simulink model "USV_SASTnewlaw_env_max"  (R2023a)
settings: Solver=ode4  StartTime=0.0  StopTime=60  FixedStep=0.01  RelTol=1e-3
undefined symbols (not defined in the file or in its folder): sigbuilder_block
libraries: sharedutil x6, simulink_extras x1, aerolibutil x1
(part 2 of 2)

== system USV_SASTnewlaw_env_max/USV_Env/Dynamic Model/Construct Matrices/M ==
  m : Inport
  X_G : Inport  Port=2
  Y_G : Inport  Port=3
  I_z : Inport  Port=4
  Hydrodynamic coefficients : Inport  Port=5
  Bus Selector : BusSelector  OutputSignals=X_u_dot,Y_r_dot,N_v_dot,Y_v_dot,N_r_dot
  Constant3 : Constant  Value=0
  Gain8 : Gain  Gain=-1
  Matrix M : sharedutil/Create 3x3 Matrix  aMode=aMode
  Product17 : Product
  Product18 : Product
  Sum14 : Sum  Inputs=|+-
  Sum15 : Sum  Inputs=+-
  Sum16 : Sum  Inputs=+-
  Sum17 : Sum  Inputs=+-
  Sum18 : Sum  Inputs=|+-
  M : Outport  VectorParamsAs1DForOutWhenUnconnected=off
  wires:
  Gain8/1 -> Matrix M/7, Matrix M/3
  Product17/1 -> Gain8/1
  Product18/1 -> Sum17/1, Sum16/1
  Sum18/1 -> Matrix M/9
  Constant3/1 -> Matrix M/4, Matrix M/2
  I_z/1 -> Sum18/1  "I_z"
  Sum15/1 -> Matrix M/5
  m/1 -> Sum14/1, Product17/1, Sum15/1, Product18/1  "m"
  Bus Selector/3 -> Sum17/2  "<N_v_dot>"
  Sum14/1 -> Matrix M/1
  Sum16/1 -> Matrix M/6
  Matrix M/1 -> M/1
  Sum17/1 -> Matrix M/8
  X_G/1 -> Product18/2  "X_G"
  Y_G/1 -> Product17/2  "Y_G"
  Bus Selector/1 -> Sum14/2  "<X_u_dot>"
  Hydrodynamic coefficients/1 -> Bus Selector/1
  Bus Selector/2 -> Sum16/2  "<Y_r_dot>"
  Bus Selector/4 -> Sum15/2  "<Y_v_dot>"
  Bus Selector/5 -> Sum18/2  "<N_r_dot>"

== system USV_SASTnewlaw_env_max/USV_Env/Dynamic Model/Construct Matrices/T-C(v)-D(v) ==
  m : Inport
  X_G : Inport  Port=2
  Y_G : Inport  Port=3
  V_Local : Inport  Port=4
  Tstbd : Inport  Port=5
  Tport : Inport  Port=6
  HydrodynamicCoefficients : Inport  Port=7
  Twind : Inport  Port=8
  Twave : Inport  Port=9
  B : Inport  Port=10
  V_r : Inport  Port=11
  C : Subsystem
  D : Subsystem
  D(v)v : Product  Multiplication=Matrix(*)
  T + Wind + Wave : Sum  Inputs=+++
  T - C(v)v - D(v)v : Sum  Inputs=+--
  Tau : Subsystem
  Out1 : Outport  VectorParamsAs1DForOutWhenUnconnected=off
  wires:
  Tstbd/1 -> Tau/2(Tstbd)
  V_r/1 -> D(v)v/2, D/2(V - r), C/6(V_r)
  T - C(v)v - D(v)v/1 -> Out1/1
  D(v)v/1 -> T - C(v)v - D(v)v/3
  B/1 -> Tau/1(B)
  C/1(C(v)v) -> T - C(v)v - D(v)v/2  "C(v)v"
  Tport/1 -> Tau/3(Tport)
  Tau/1(T) -> T + Wind + Wave/1
  D/1(D(v)) -> D(v)v/1  "D(v)"
  HydrodynamicCoefficients/1 -> C/4(Hydrodynamic coefficients), D/1(Hydrodynamic Coefficients)
  Y_G/1 -> C/3(Y_G)
  X_G/1 -> C/2(X_G)
  m/1 -> C/1(m)
  T + Wind + Wave/1 -> T - C(v)v - D(v)v/1
  Twind/1 -> T + Wind + Wave/2
  Twave/1 -> T + Wind + Wave/3
  V_Local/1 -> C/5(V local)

== system USV_SASTnewlaw_env_max/USV_Env/Waves/Fwave/w ==
  Demux : Demux  Tag=STV Demux  Outputs=3
      settings: DisplayOption=none
  FromWs : FromWorkspace  Tag=STV FromWs  VariableName=tuvar
      SigBuilderData=|
      | common.afterFinalStr = 'Extrapolate'
      | common.sampleTime = 0
      | dataSet.timeRange = [0 200]
      | dataSet.name = 'Group 1'
      | sbobj.Groups.Name = 'Group 1'
      | sbobj.Groups.Signals(1).Name = 'w'
      | sbobj.Groups.Signals(1).XData = [0 0.05 0.1 0.15 0.2 0.25 0.3 0.35 0.4 0.45 0.5 0.55 ... (4001 elements, 1x4001)]
      | sbobj.Groups.Signals(1).YData = [5.37667139546 18.338850146 -22.58846861 8.62173320368 3.18765239859 -13.0768829631 -4.33592022306 3.42624466539 35.7839693973 27.6943702988 -13.4988694016 30.3492346633 ... (4001 elements, 1x4001)]
      | sbobj.Groups.Signals(2).Name = 'd'
      | sbobj.Groups.Signals(2).XData = [0 0.05 0.1 0.15 0.2 0.25 0.3 0.35 0.4 0.45 0.5 0.55 ... (4001 elements, 1x4001)]
      | sbobj.Groups.Signals(2).YData = [1.96793906261 -2.502772713 -0.359507581211 -1.48681289659 0.466483843385 4.20268960924 -1.75333262292 3.8975770962 -0.930544368142 -1.30383439898 1.21926117699 1.41824803192 ... (4001 elements, 1x4001)]
      | sbobj.Groups.Signals(3).Name = 'zero'
      | sbobj.Groups.Signals(3).XData = [0 200]
      | sbobj.Groups.Signals(3).YData = [0 0]
      | sbobj.Groups.TimeRange = [0 200]
  w : Outport  Tag=STV Outport
  d : Outport  Tag=STV Outport  Port=2
  zero : Outport  Tag=STV Outport  Port=3
  wires:
  Demux/1 -> w/1
  FromWs/1 -> Demux/1
  Demux/2 -> d/1
  Demux/3 -> zero/1

== system USV_SASTnewlaw_env_max/USV_Env/Waves/N/w ==
  Demux : Demux  Tag=STV Demux  Outputs=3
      settings: DisplayOption=none
  FromWs : FromWorkspace  Tag=STV FromWs  VariableName=tuvar
      SigBuilderData=|
      | common.afterFinalStr = 'Extrapolate'
      | common.sampleTime = 0
      | dataSet.timeRange = [0 200]
      | dataSet.name = 'Group 1'
      | sbobj.Groups.Name = 'Group 1'
      | sbobj.Groups.Signals(1).Name = 'w'
      | sbobj.Groups.Signals(1).XData = [0 0.05 0.1 0.15 0.2 0.25 0.3 0.35 0.4 0.45 0.5 0.55 ... (4001 elements, 1x4001)]
      | sbobj.Groups.Signals(1).YData = [1.00042183788 -0.588063687899 1.55748343179 -1.36137320604 1.90008161512 0.177859224675 -2.16660961344 0.706892217353 -2.22533446552 0.34119917378 2.25123807911 -0.166136696753 ... (4001 elements, 1x4001)]
      | sbobj.Groups.Signals(2).Name = 'd'
      | sbobj.Groups.Signals(2).XData = [0 0.05 0.1 0.15 0.2 0.25 0.3 0.35 0.4 0.45 0.5 0.55 ... (4001 elements, 1x4001)]
      | sbobj.Groups.Signals(2).YData = [-0.0589712527229 0.138137750494 -0.0304333425469 0.019542517604 0.115882491211 0.00329758407129 -0.0955163588139 -0.0273105595941 0.115777992108 -0.0703785233673 0.114116406605 -0.0158128154965 ... (4001 elements, 1x4001)]
      | sbobj.Groups.Signals(3).Name = 'zero'
      | sbobj.Groups.Signals(3).XData = [0 200]
      | sbobj.Groups.Signals(3).YData = [0 0]
      | sbobj.Groups.TimeRange = [0 200]
  w : Outport  Tag=STV Outport
  d : Outport  Tag=STV Outport  Port=2
  zero : Outport  Tag=STV Outport  Port=3
  wires:
  Demux/1 -> w/1
  FromWs/1 -> Demux/1
  Demux/2 -> d/1
  Demux/3 -> zero/1

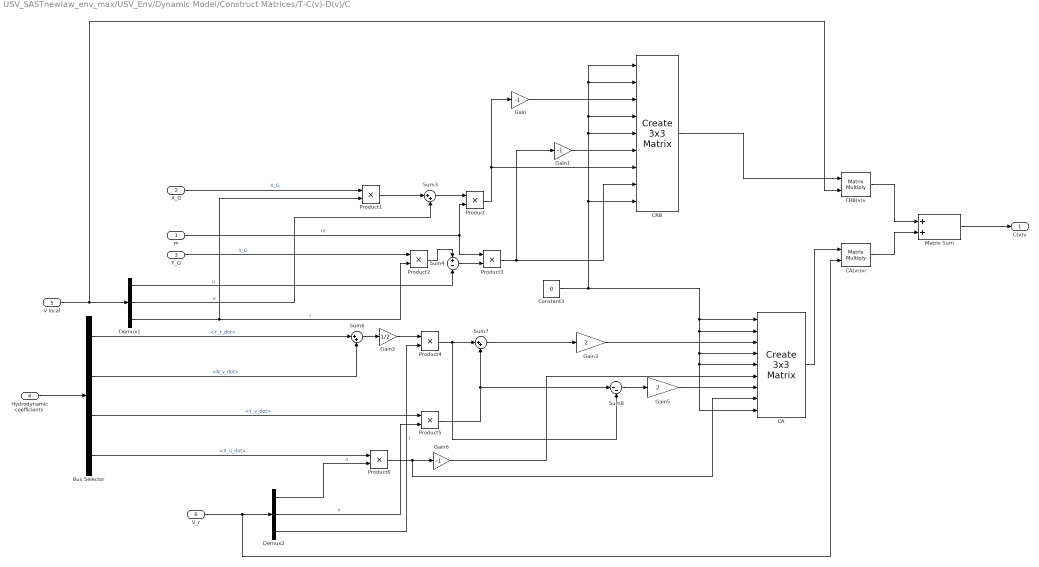
== system USV_SASTnewlaw_env_max/USV_Env/Dynamic Model/Construct Matrices/T-C(v)-D(v)/C ==
  m : Inport
  X_G : Inport  Port=2
  Y_G : Inport  Port=3
  Hydrodynamic coefficients : Inport  Port=4
  V local : Inport  Port=5
  V_r : Inport  Port=6
  " CRB" : sharedutil/Create 3x3 Matrix  aMode=aMode
  Bus Selector : BusSelector  OutputSignals=Y_r_dot,N_v_dot,Y_v_dot,X_u_dot
  CA : sharedutil/Create 3x3 Matrix  aMode=aMode
  CA(vr)vr : Product  Multiplication=Matrix(*)
  CRB(v)v : Product  Multiplication=Matrix(*)
  Constant3 : Constant  Value=0
  Demux1 : Demux  Outputs=3
  Demux2 : Demux  Outputs=3
  Gain : Gain  Gain=-1
  Gain1 : Gain  Gain=-1
  Gain2 : Gain  Gain=1/2
  Gain3 : Gain  Gain=2
  Gain5 : Gain  Gain=2
  Gain6 : Gain  Gain=-1
  Matrix Sum : Sum
  Product{,1..6} (7 alike) : Product
  Sum3 : Sum  Inputs=|++
  Sum4 : Sum  Inputs=+-
  Sum6 : Sum  Inputs=|++
  Sum7 : Sum  Inputs=|++
  Sum8 : Sum  Inputs=|--
  C(v)v : Outport  VectorParamsAs1DForOutWhenUnconnected=off
  wires:
  Bus Selector/1 -> Sum6/1  "<Y_r_dot>"
  Demux1/3 -> Product1/2, Product2/2  "r"
  Gain2/1 -> Product4/1
  CA/1 -> CA(vr)vr/1
  Gain/1 -> " CRB"/3
  Bus Selector/2 -> Sum6/2  "<N_v_dot>"
  Sum3/1 -> Product/1
  Sum8/1 -> Gain5/1
  Product2/1 -> Sum4/1
  Sum6/1 -> Gain2/1
  Product5/1 -> Sum7/2, Sum8/1
  Gain1/1 -> " CRB"/6
  Product1/1 -> Sum3/1
  Y_G/1 -> Product2/1  "Y_G"
  Matrix Sum/1 -> C(v)v/1
  Gain3/1 -> CA/3
  Gain6/1 -> CA/6
  Product6/1 -> Gain6/1, CA/8
  Demux1/2 -> Sum3/2  "v"
  Product4/1 -> Sum7/1, Sum8/2
  Product3/1 -> " CRB"/8, Gain1/1
  Gain5/1 -> CA/7
  " CRB"/1 -> CRB(v)v/1
  X_G/1 -> Product1/1  "X_G"
  Sum7/1 -> Gain3/1
  Product/1 -> " CRB"/7, Gain/1
  m/1 -> Product/2, Product3/1  "m"
  Constant3/1 -> " CRB"/5, " CRB"/4, " CRB"/2, " CRB"/1, " CRB"/9, CA/4, CA/5, CA/9, CA/2, CA/1
  Hydrodynamic coefficients/1 -> Bus Selector/1
  Bus Selector/4 -> Product6/1  "<X_u_dot>"
  Bus Selector/3 -> Product5/1  "<Y_v_dot>"
  Demux1/1 -> Sum4/2  "u"
  V local/1 -> CRB(v)v/2, Demux1/1
  Sum4/1 -> Product3/2
  V_r/1 -> CA(vr)vr/2, Demux2/1
  CA(vr)vr/1 -> Matrix Sum/2
  CRB(v)v/1 -> Matrix Sum/1
  Demux2/1 -> Product6/2  "u"
  Demux2/2 -> Product5/2  "v"
  Demux2/3 -> Product4/2  "r"

== system USV_SASTnewlaw_env_max/USV_Env/Dynamic Model/Construct Matrices/T-C(v)-D(v)/D ==
  Hydrodynamic Coefficients : Inport
  V - r : Inport  Port=2
  Abs r : Abs  SaturateOnIntegerOverflow=off
  Abs u : Abs  SaturateOnIntegerOverflow=off
  Abs v : Abs  SaturateOnIntegerOverflow=off
  Bus Selector : BusSelector  OutputSignals=X_u,Y_v,Y_r,X_u|u|,Y_v|v|,Y_v|r|,Y_r|v|,N_v,N_r,Y_r|r|,N_v|v|,N_v|r|,N_r|r|,N_r|v|
  Constant : Constant  Value=0
  D : Sum
  Demux : Demux  Outputs=3
  Dl : sharedutil/Create 3x3 Matrix  aMode=aMode
  Dn : sharedutil/Create 3x3 Matrix  aMode=aMode
  Gain4 : Gain  Gain=-1
  Gain7 : Gain  Gain=-1
  Product7 : Product
  Subsystem : Subsystem
  Subsystem1 : Subsystem
  Subsystem2 : Subsystem
  Subsystem3 : Subsystem
  D(v) : Outport  VectorParamsAs1DForOutWhenUnconnected=off
  wires:
  Constant/1 -> Dn/7, Dn/4, Dn/3, Dn/2, Dl/7, Dl/4, Dl/3, Dl/2
  Abs u/1 -> Product7/2
  Abs r/1 -> Subsystem/3(Abs_r), Subsystem3/2("Abs_r "), Subsystem2/2(Abs_r), Subsystem1/1(Abs_r)  "Abs_r"
  Product7/1 -> Dn/1
  Abs v/1 -> Subsystem/4("Abs_v "), Subsystem3/4(Abs_v), Subsystem1/4(Abs_v), Subsystem2/4(Abs_v)  "Abs_v"
  Gain7/1 -> D/2
  Gain4/1 -> D/1
  Dl/1 -> Gain4/1
  Dn/1 -> Gain7/1
  D/1 -> D(v)/1
  Subsystem/1(Out1) -> Dn/5
  Subsystem1/1(Out1) -> Dn/9
  Subsystem2/1(Out1) -> Dn/8
  Subsystem3/1(Out1) -> Dn/6
  Hydrodynamic Coefficients/1 -> Bus Selector/1
  Bus Selector/5 -> Subsystem/1("Y_v|v| ")  "<Y_v|v|>"
  Bus Selector/6 -> Subsystem/2(Y_v|r|)  "<Y_v|r|>"
  Bus Selector/2 -> Dl/5  "<Y_v>"
  Bus Selector/7 -> Subsystem3/1(Y_r|v|)  "<Y_r|v|>"
  Bus Selector/10 -> Subsystem3/3(Y_r|r|)  "<Y_r|r|>"
  Bus Selector/11 -> Subsystem2/3(N_v|v|)  "<N_v|v|>"
  Bus Selector/8 -> Dl/8  "<N_v>"
  Bus Selector/12 -> Subsystem2/1(N_v|r|)  "<N_v|r|>"
  Bus Selector/14 -> Subsystem1/3(N_r|v|)  "<N_r|v|>"
  Bus Selector/9 -> Dl/9  "<N_r>"
  Bus Selector/13 -> Subsystem1/2(N_r|r|)  "<N_r|r|>"
  Bus Selector/1 -> Dl/1  "<X_u>"
  Bus Selector/4 -> Product7/1  "<X_u|u|>"
  Bus Selector/3 -> Dl/6  "<Y_r>"
  Demux/1 -> Abs u/1  "u"
  Demux/2 -> Abs v/1  "v"
  Demux/3 -> Abs r/1  "r"
  V - r/1 -> Demux/1

== system USV_SASTnewlaw_env_max/USV_Env/Dynamic Model/Construct Matrices/T-C(v)-D(v)/Tau ==
  B : Inport
  Tstbd : Inport  Port=2
  Tport : Inport  Port=3
  Mux : Mux  Inputs=3
  Product25 : Product
  Sum : Sum  Inputs=|++
  Sum1 : Sum  Inputs=|+-
  Ty : Constant  Value=0
  Tz : Gain  Gain=1/2
  T : Outport  VectorParamsAs1DForOutWhenUnconnected=off
  wires:
  Product25/1 -> Tz/1
  Tz/1 -> Mux/3  "Tz"
  Mux/1 -> T/1  "T"
  B/1 -> Product25/2  "B"
  Sum1/1 -> Product25/1
  Ty/1 -> Mux/2  "Ty"
  Tstbd/1 -> Sum/2, Sum1/2  "Tstbd"
  Tport/1 -> Sum/1, Sum1/1  "Tport"
  Sum/1 -> Mux/1

== system USV_SASTnewlaw_env_max/USV_Env/Dynamic Model/Construct Matrices/T-C(v)-D(v)/D/Subsystem ==
  "Y_v|v| " : Inport
  Y_v|r| : Inport  Port=2
  Abs_r : Inport  Port=3
  "Abs_v " : Inport  Port=4
  Product8 : Product
  Product9 : Product
  Sum10 : Sum  Inputs=|++
  Out1 : Outport  VectorParamsAs1DForOutWhenUnconnected=off
  wires:
  Y_v|r|/1 -> Product9/1
  Abs_r/1 -> Product9/2
  Product9/1 -> Sum10/2
  "Y_v|v| "/1 -> Product8/1
  Product8/1 -> Sum10/1
  "Abs_v "/1 -> Product8/2
  Sum10/1 -> Out1/1

== system USV_SASTnewlaw_env_max/USV_Env/Dynamic Model/Construct Matrices/T-C(v)-D(v)/D/Subsystem1 ==
  Abs_r : Inport
  N_r|r| : Inport  Port=2
  N_r|v| : Inport  Port=3
  Abs_v : Inport  Port=4
  Product14 : Product
  Product15 : Product
  Sum13 : Sum  Inputs=|++
  Out1 : Outport  VectorParamsAs1DForOutWhenUnconnected=off
  wires:
  Product15/1 -> Sum13/1
  Sum13/1 -> Out1/1
  N_r|v|/1 -> Product14/1
  Product14/1 -> Sum13/2
  Abs_r/1 -> Product15/2
  N_r|r|/1 -> Product15/1
  Abs_v/1 -> Product14/2

== system USV_SASTnewlaw_env_max/USV_Env/Dynamic Model/Construct Matrices/T-C(v)-D(v)/D/Subsystem2 ==
  N_v|r| : Inport
  Abs_r : Inport  Port=2
  N_v|v| : Inport  Port=3
  Abs_v : Inport  Port=4
  Product12 : Product
  Product13 : Product
  Sum12 : Sum  Inputs=|++
  Out1 : Outport  VectorParamsAs1DForOutWhenUnconnected=off
  wires:
  Sum12/1 -> Out1/1
  Product13/1 -> Sum12/1
  N_v|v|/1 -> Product12/1
  Product12/1 -> Sum12/2
  Abs_r/1 -> Product13/2
  Abs_v/1 -> Product12/2
  N_v|r|/1 -> Product13/1

== system USV_SASTnewlaw_env_max/USV_Env/Dynamic Model/Construct Matrices/T-C(v)-D(v)/D/Subsystem3 ==
  Y_r|v| : Inport
  "Abs_r " : Inport  Port=2
  Y_r|r| : Inport  Port=3
  Abs_v : Inport  Port=4
  Product10 : Product
  Product11 : Product
  Sum11 : Sum  Inputs=|++
  Out1 : Outport  VectorParamsAs1DForOutWhenUnconnected=off
  wires:
  Product11/1 -> Sum11/2
  Product10/1 -> Sum11/1
  Sum11/1 -> Out1/1
  Y_r|v|/1 -> Product10/1
  "Abs_r "/1 -> Product11/2
  Y_r|r|/1 -> Product11/1
  Abs_v/1 -> Product10/2

== matlab function USV_SASTnewlaw_env_max/track/yddot_d ==
  data: yddot_d input; l input; psid input; rd input; yddot output; rdot_d input
function yddot   = fcn(yddot_d, l, psid, rd, rdot_d)
yddot = yddot_d + l*cos(psid)*rdot_d - l*sin(psid)*rd*rd;

== matlab function USV_SASTnewlaw_env_max/track/tracking_ctrl ==
  data: u input; v input; r input; psi input; tu output; fu input; gu input; fv input; fr input; gr input; uax input; uay input; le2x input; le2y input; tr output; l input; xddot_d input; yddot_d input
function [tu,tr]  = fcn(u, v, r, psi, fu, gu, fv, fr, gr, uax, uay, le2x, le2y, l, xddot_d, yddot_d)
gz = [gu*cos(psi), -gr*l*sin(psi); gu*sin(psi), gr*l*cos(psi)];
lep = [le2x; le2y];
f1 = [cos(psi), -sin(psi); sin(psi), cos(psi)];
f2 = [fu - v*r - l*r*r; u*r + fv + l*fr];
fz = f1*f2;
ua = [uax; uay];
ref_ddot = [xddot_d; yddot_d];
uz = inv(gz)*(ref_ddot + lep - fz - ua);
tu = uz(1);
tr = uz(2);

== matlab function USV_SASTnewlaw_env_max/track/xdot ==
  data: u input; v input; r input; psi input; xdot output; l input
function xdot   = fcn(u, v, r, psi, l)
xdot = u*cos(psi)-v*sin(psi)-r*l*sin(psi);

== matlab function USV_SASTnewlaw_env_max/track/ydot ==
  data: u input; v input; r input; psi input; ydot output; l input
function ydot   = fcn(u, v, r, psi, l)
ydot = u*sin(psi)+v*cos(psi)+r*l*cos(psi);

== matlab function USV_SASTnewlaw_env_max/track/xdot_d ==
  data: xdot_d input; l input; psid input; rd input; xdot output
function xdot   = fcn(xdot_d, l, psid, rd)
xdot = xdot_d - l*sin(psid)*rd;

== matlab function USV_SASTnewlaw_env_max/track/ydot_d ==
  data: ydot_d input; l input; psid input; rd input; ydot output
function ydot   = fcn(ydot_d, l, psid, rd)
ydot = ydot_d + l*cos(psid)*rd;

== matlab function USV_SASTnewlaw_env_max/track/xddot_d ==
  data: xddot_d input; l input; psid input; rd input; xddot output; rdot_d input
function xddot   = fcn(xddot_d, l, psid, rd, rdot_d)
xddot = xddot_d - l*sin(psid)*rdot_d - l*cos(psid)*rd*rd;
